simulink model "SoftRobot_AdaptivePassivity_FaultObserver_Tracking_S3"  (R2021b)
settings: Solver=FixedStepAuto  StartTime=0.0  StopTime=30  FixedStep=0.001  RelTol=1e-3  EnableMultiTasking=on
libraries: simulink x3
(part 2 of 2)

== matlab function SoftRobot_AdaptivePassivity_FaultObserver_Tracking_S3/Sliding mode variable//LIP form//Adaptation law ==
  data: Y output; q input; q_dot input; q_des input; theta_hat_dot output; q_dot_des input; q_dotdot_des input; lambda input; adaptation_rate input; r output
function [Y,theta_hat_dot,r] = fcn(q,q_dot,q_des,q_dot_des,q_dotdot_des,lambda,adaptation_rate)

l1=0.067;
l2=0.077;

q1 = q(1);
q2 = q(2);
q_dot1 = q_dot(1);
q_dot2 = q_dot(2);

v = q_dot_des-lambda*(q-q_des);
v1 = v(1);
v2 = v(2);

v_dot = q_dotdot_des-lambda*(q_dot-q_dot_des);
v_dot1 = v_dot(1);
v_dot2 = v_dot(2);

Y1 = [((981*l1*q2*sin(q1))/200 - (981*l1*q1*q2*cos(q1))/200)/(q1^2*q2) - v1*((q_dot2*((2*((l1^2*q2^2)/2 + (l1^2*q1^2*q2^2)/4 - (l1^2*q2^2*cos(q1))/2 - (l1^2*q1*q2^2*sin(q1))/2))/(q1^4*q2^3) - (l1^2*q2 + (l1^2*q1^2*q2)/2 - l1^2*q2*cos(q1) - l1^2*q1*q2*sin(q1))/(q1^4*q2^2)))/2 - (q_dot1*(((l1^2*q1*q2^2)/2 - (l1^2*q1*q2^2*cos(q1))/2)/(q1^4*q2^2) - (4*((l1^2*q2^2)/2 + (l1^2*q1^2*q2^2)/4 - (l1^2*q2^2*cos(q1))/2 - (l1^2*q1*q2^2*sin(q1))/2))/(q1^5*q2^2)))/2) + (v_dot1*((l1^2*q2^2)/2 + (l1^2*q1^2*q2^2)/4 - (l1^2*q2^2*cos(q1))/2 - (l1^2*q1*q2^2*sin(q1))/2))/(q1^4*q2^2), ((981*l1*q2*sin(q1))/100 - (981*l1*q1*q2*cos(q1))/100)/(q1^2*q2) - v1*((q_dot2*((2*(2*l1^2*q2^2 + l1^2*q1^2*q2^2 - 2*l1^2*q2^2*cos(q1) - 2*l1^2*q1*q2^2*sin(q1)))/(q1^4*q2^3) - (4*l1^2*q2 + 2*l1^2*q1^2*q2 - 4*l1^2*q2*cos(q1) - 4*l1^2*q1*q2*sin(q1))/(q1^4*q2^2)))/2 - (q_dot1*((2*l1^2*q1*q2^2 - 2*l1^2*q1*q2^2*cos(q1))/(q1^4*q2^2) - (4*(2*l1^2*q2^2 + l1^2*q1^2*q2^2 - 2*l1^2*q2^2*cos(q1) - 2*l1^2*q1*q2^2*sin(q1)))/(q1^5*q2^2)))/2) + (v_dot1*(2*l1^2*q2^2 + l1^2*q1^2*q2^2 - 2*l1^2*q2^2*cos(q1) - 2*l1^2*q1*q2^2*sin(q1)))/(q1^4*q2^2), ((981*l1*q2*sin(q1))/100 - (981*l1*q1*q2*cos(q1))/100)/(q1^2*q2) - v1*((q_dot2*((2*(2*l1^2*q2^2 + l1^2*q1^2*q2^2 - 2*l1^2*q2^2*cos(q1) - 2*l1^2*q1*q2^2*sin(q1)))/(q1^4*q2^3) - (4*l1^2*q2 + 2*l1^2*q1^2*q2 - 4*l1^2*q2*cos(q1) - 4*l1^2*q1*q2*sin(q1))/(q1^4*q2^2)))/2 - (q_dot1*((2*l1^2*q1*q2^2 - 2*l1^2*q1*q2^2*cos(q1))/(q1^4*q2^2) - (4*(2*l1^2*q2^2 + l1^2*q1^2*q2^2 - 2*l1^2*q2^2*cos(q1) - 2*l1^2*q1*q2^2*sin(q1)))/(q1^5*q2^2)))/2) + (v_dot1*(2*l1^2*q2^2 + l1^2*q1^2*q2^2 - 2*l1^2*q2^2*cos(q1) - 2*l1^2*q1*q2^2*sin(q1)))/(q1^4*q2^2), ((981*l1*q2*sin(q1))/100 - (981*l2*q1^2*cos(q1 + q2))/200 + (981*l2*q1^2*cos(q1))/200 - (981*l1*q1*q2*cos(q1))/100)/(q1^2*q2) - v1*((q_dot1*((4*(2*l1^2*q2^2 + (l2^2*q1^4)/2 + l1^2*q1^2*q2^2 - 2*l1^2*q2^2*cos(q1) - (l2^2*q1^4*cos(q2))/2 - 2*l1^2*q1*q2^2*sin(q1) - l1*l2*q1^3*q2 - l1*l2*q1^2*q2*sin(q1 + q2) + l1*l2*q1^3*q2*cos(q2) + l1*l2*q1^2*q2*sin(q1) + l1*l2*q1^2*q2*sin(q2)))/(q1^5*q2^2) - (2*l2^2*q1^3 + 2*l1^2*q1*q2^2 - 2*l2^2*q1^3*cos(q2) - 2*l1^2*q1*q2^2*cos(q1) - 3*l1*l2*q1^2*q2 - l1*l2*q1^2*q2*cos(q1 + q2) + l1*l2*q1^2*q2*cos(q1) + 3*l1*l2*q1^2*q2*cos(q2) - 2*l1*l2*q1*q2*sin(q1 + q2) + 2*l1*l2*q1*q2*sin(q1) + 2*l1*l2*q1*q2*sin(q2))/(q1^4*q2^2)))/2 + (q_dot2*((2*(2*l1^2*q2^2 + (l2^2*q1^4)/2 + l1^2*q1^2*q2^2 - 2*l1^2*q2^2*cos(q1) - (l2^2*q1^4*cos(q2))/2 - 2*l1^2*q1*q2^2*sin(q1) - l1*l2*q1^3*q2 - l1*l2*q1^2*q2*sin(q1 + q2) + l1*l2*q1^3*q2*cos(q2) + l1*l2*q1^2*q2*sin(q1) + l1*l2*q1^2*q2*sin(q2)))/(q1^4*q2^3) - (4*l1^2*q2 - l1*l2*q1^3 + 2*l1^2*q1^2*q2 - 4*l1^2*q2*cos(q1) + (l2^2*q1^4*sin(q2))/2 - l1*l2*q1^2*sin(q1 + q2) + l1*l2*q1^3*cos(q2) + l1*l2*q1^2*sin(q1) + l1*l2*q1^2*sin(q2) - 4*l1^2*q1*q2*sin(q1) - l1*l2*q1^2*q2*cos(q1 + q2) + l1*l2*q1^2*q2*cos(q2) - l1*l2*q1^3*q2*sin(q2))/(q1^4*q2^2)))/2) + (v_dot1*(2*l1^2*q2^2 + (l2^2*q1^4)/2 + l1^2*q1^2*q2^2 - 2*l1^2*q2^2*cos(q1) - (l2^2*q1^4*cos(q2))/2 - 2*l1^2*q1*q2^2*sin(q1) - l1*l2*q1^3*q2 - l1*l2*q1^2*q2*sin(q1 + q2) + l1*l2*q1^3*q2*cos(q2) + l1*l2*q1^2*q2*sin(q1) + l1*l2*q1^2*q2*sin(q2)))/(q1^4*q2^2) - (l2*v2*(2*l2*q1^2*q_dot1 - 4*l1*q_dot2 + 2*l2*q1^2*q_dot2 + 4*l1*q_dot2*cos(q1) + 4*l1*q_dot2*cos(q2) - 4*l1*q_dot2*cos(q1 + q2) - 2*l1*q1*q2*q_dot1 - 2*l1*q2*q_dot1*sin(q1 + q2) - 4*l1*q2*q_dot2*sin(q1 + q2) + 2*l1*q2*q_dot1*sin(q1) - 4*l1*q1*q_dot2*sin(q2) + 2*l1*q2*q_dot1*sin(q2) + 4*l1*q2*q_dot2*sin(q2) + 2*l1*q2^2*q_dot1*cos(q1 + q2) + 2*l1*q2^2*q_dot2*cos(q1 + q2) - 2*l1*q2^2*q_dot1*cos(q2) - 2*l2*q1^2*q_dot1*cos(q2) - 2*l1*q2^2*q_dot2*cos(q2) - 2*l2*q1^2*q_dot2*cos(q2) + 2*l1*q1*q2^2*q_dot1*sin(q2) + 2*l1*q1*q2^2*q_dot2*sin(q2) - l2*q1^2*q2*q_dot1*sin(q2) - l2*q1^2*q2*q_dot2*sin(q2) + 2*l1*q1*q2*q_dot1*cos(q2) + 4*l1*q1*q2*q_dot2*cos(q2)))/(4*q1^2*q2^3) - (l2*v_dot2*(2*l1 + 2*l1*cos(q1 + q2) - l2*q1^2 - 2*l1*cos(q1) - 2*l1*cos(q2) + 2*l1*q1*sin(q2) - 2*l1*q2*sin(q2) + l2*q1^2*cos(q2) + 2*l1*q2*sin(q1 + q2) - 2*l1*q1*q2*cos(q2)))/(4*q1^2*q2^2), ((981*l1*q2*sin(q1))/100 - (981*l2*q1^2*cos(q1 + q2))/100 + (981*l2*q1^2*cos(q1))/100 - (981*l1*q1*q2*cos(q1))/100)/(q1^2*q2) - v1*((q_dot1*((4*(2*l1^2*q2^2 + 2*l2^2*q1^4 + l1^2*q1^2*q2^2 - 2*l1^2*q2^2*cos(q1) - 2*l2^2*q1^4*cos(q2) - 2*l1^2*q1*q2^2*sin(q1) - 2*l1*l2*q1^3*q2 - 2*l1*l2*q1^2*q2*sin(q1 + q2) + 2*l1*l2*q1^3*q2*cos(q2) + 2*l1*l2*q1^2*q2*sin(q1) + 2*l1*l2*q1^2*q2*sin(q2)))/(q1^5*q2^2) - (8*l2^2*q1^3 + 2*l1^2*q1*q2^2 - 8*l2^2*q1^3*cos(q2) - 2*l1^2*q1*q2^2*cos(q1) - 6*l1*l2*q1^2*q2 - 2*l1*l2*q1^2*q2*cos(q1 + q2) + 2*l1*l2*q1^2*q2*cos(q1) + 6*l1*l2*q1^2*q2*cos(q2) - 4*l1*l2*q1*q2*sin(q1 + q2) + 4*l1*l2*q1*q2*sin(q1) + 4*l1*l2*q1*q2*sin(q2))/(q1^4*q2^2)))/2 + (q_dot2*((2*(2*l1^2*q2^2 + 2*l2^2*q1^4 + l1^2*q1^2*q2^2 - 2*l1^2*q2^2*cos(q1) - 2*l2^2*q1^4*cos(q2) - 2*l1^2*q1*q2^2*sin(q1) - 2*l1*l2*q1^3*q2 - 2*l1*l2*q1^2*q2*sin(q1 + q2) + 2*l1*l2*q1^3*q2*cos(q2) + 2*l1*l2*q1^2*q2*sin(q1) + 2*l1*l2*q1^2*q2*sin(q2)))/(q1^4*q2^3) - (4*l1^2*q2 - 2*l1*l2*q1^3 + 2*l1^2*q1^2*q2 - 4*l1^2*q2*cos(q1) + 2*l2^2*q1^4*sin(q2) - 2*l1*l2*q1^2*sin(q1 + q2) + 2*l1*l2*q1^3*cos(q2) + 2*l1*l2*q1^2*sin(q1) + 2*l1*l2*q1^2*sin(q2) - 4*l1^2*q1*q2*sin(q1) - 2*l1*l2*q1^2*q2*cos(q1 + q2) + 2*l1*l2*q1^2*q2*cos(q2) - 2*l1*l2*q1^3*q2*sin(q2))/(q1^4*q2^2)))/2) + (v_dot1*(2*l1^2*q2^2 + 2*l2^2*q1^4 + l1^2*q1^2*q2^2 - 2*l1^2*q2^2*cos(q1) - 2*l2^2*q1^4*cos(q2) - 2*l1^2*q1*q2^2*sin(q1) - 2*l1*l2*q1^3*q2 - 2*l1*l2*q1^2*q2*sin(q1 + q2) + 2*l1*l2*q1^3*q2*cos(q2) + 2*l1*l2*q1^2*q2*sin(q1) + 2*l1*l2*q1^2*q2*sin(q2)))/(q1^4*q2^2) - (l2*v2*(8*l2*q1^2*q_dot1 - 8*l1*q_dot2 + 8*l2*q1^2*q_dot2 + 8*l1*q_dot2*cos(q1) + 8*l1*q_dot2*cos(q2) - 8*l1*q_dot2*cos(q1 + q2) - 4*l1*q1*q2*q_dot1 - 4*l1*q2*q_dot1*sin(q1 + q2) - 8*l1*q2*q_dot2*sin(q1 + q2) + 4*l1*q2*q_dot1*sin(q1) - 8*l1*q1*q_dot2*sin(q2) + 4*l1*q2*q_dot1*sin(q2) + 8*l1*q2*q_dot2*sin(q2) + 4*l1*q2^2*q_dot1*cos(q1 + q2) + 4*l1*q2^2*q_dot2*cos(q1 + q2) - 4*l1*q2^2*q_dot1*cos(q2) - 8*l2*q1^2*q_dot1*cos(q2) - 4*l1*q2^2*q_dot2*cos(q2) - 8*l2*q1^2*q_dot2*cos(q2) + 4*l1*q1*q2^2*q_dot1*sin(q2) + 4*l1*q1*q2^2*q_dot2*sin(q2) - 4*l2*q1^2*q2*q_dot1*sin(q2) - 4*l2*q1^2*q2*q_dot2*sin(q2) + 4*l1*q1*q2*q_dot1*cos(q2) + 8*l1*q1*q2*q_dot2*cos(q2)))/(4*q1^2*q2^3) - (l2*v_dot2*(4*l1 + 4*l1*cos(q1 + q2) - 4*l2*q1^2 - 4*l1*cos(q1) - 4*l1*cos(q2) + 4*l1*q1*sin(q2) - 4*l1*q2*sin(q2) + 4*l2*q1^2*cos(q2) + 4*l1*q2*sin(q1 + q2) - 4*l1*q1*q2*cos(q2)))/(4*q1^2*q2^2), q1, v1];
Y2 = [(q_dot2*v2*((l2^2*(2*cos(q2) + 2*q2*sin(q2) - q2^2 - 2))/q2^5 + (l2^2*(2*q2 - 2*q2*cos(q2)))/(4*q2^4)))/2 - (981*l2*(sin(q1) - sin(q1 + q2) + q2*cos(q1 + q2)))/(200*q2^2) - (l2^2*v_dot2*(2*cos(q2) + 2*q2*sin(q2) - q2^2 - 2))/(4*q2^4) - (l2*v_dot1*(2*l1 + 2*l1*cos(q1 + q2) - l2*q1^2 - 2*l1*cos(q1) - 2*l1*cos(q2) + 2*l1*q1*sin(q2) - 2*l1*q2*sin(q2) + l2*q1^2*cos(q2) + 2*l1*q2*sin(q1 + q2) - 2*l1*q1*q2*cos(q2)))/(4*q1^2*q2^2) + (l2*q_dot1*v1*(4*l1*q2 + 2*l2*q1^3 - 2*l1*q1^2*q2 - 4*l1*q2*cos(q1) - 4*l1*q2*cos(q2) + 4*l1*q2^2*sin(q1 + q2) - 2*l2*q1^3*cos(q2) - 4*l1*q2^2*sin(q2) + 4*l1*q2*cos(q1 + q2) + 2*l1*q1^2*q2^2*sin(q2) + 4*l1*q1*q2*sin(q2) - 4*l1*q1*q2^2*cos(q2) + 2*l1*q1^2*q2*cos(q2) - l2*q1^3*q2*sin(q2)))/(4*q1^3*q2^3), (q_dot2*v2*((4*l2^2*(2*cos(q2) + 2*q2*sin(q2) - q2^2 - 2))/q2^5 + (l2^2*(2*q2 - 2*q2*cos(q2)))/q2^4))/2 - (981*l2*(sin(q1) - sin(q1 + q2) + q2*cos(q1 + q2)))/(100*q2^2) - (l2^2*v_dot2*(2*cos(q2) + 2*q2*sin(q2) - q2^2 - 2))/q2^4 - (l2*v_dot1*(4*l1 + 4*l1*cos(q1 + q2) - 4*l2*q1^2 - 4*l1*cos(q1) - 4*l1*cos(q2) + 4*l1*q1*sin(q2) - 4*l1*q2*sin(q2) + 4*l2*q1^2*cos(q2) + 4*l1*q2*sin(q1 + q2) - 4*l1*q1*q2*cos(q2)))/(4*q1^2*q2^2) + (l2*q_dot1*v1*(8*l1*q2 + 8*l2*q1^3 - 4*l1*q1^2*q2 - 8*l1*q2*cos(q1) - 8*l1*q2*cos(q2) + 8*l1*q2^2*sin(q1 + q2) - 8*l2*q1^3*cos(q2) - 8*l1*q2^2*sin(q2) + 8*l1*q2*cos(q1 + q2) + 4*l1*q1^2*q2^2*sin(q2) + 8*l1*q1*q2*sin(q2) - 8*l1*q1*q2^2*cos(q2) + 4*l1*q1^2*q2*cos(q2) - 4*l2*q1^3*q2*sin(q2)))/(4*q1^3*q2^3), q2, v2];
Y = blkdiag(Y1,Y2);

% Y=[ -(l1*(981*q1^4*cos(q1) - 981*q1^3*sin(q1) - 50*l1*q1^3*v_dot1 - 100*l1*q1*v_dot1 + 200*l1*q_dot1*v1 + 50*l1*q1^2*q_dot1*v1 + 100*l1*q1*v_dot1*cos(q1) - 200*l1*q_dot1*v1*cos(q1) + 100*l1*q1^2*v_dot1*sin(q1) - 200*l1*q1*q_dot1*v1*sin(q1) + 50*l1*q1^2*q_dot1*v1*cos(q1)))/(200*q1^5), -(l1*(981*q1^4*cos(q1) - 981*q1^3*sin(q1) - 100*l1*q1^3*v_dot1 - 200*l1*q1*v_dot1 + 400*l1*q_dot1*v1 + 100*l1*q1^2*q_dot1*v1 + 200*l1*q1*v_dot1*cos(q1) - 400*l1*q_dot1*v1*cos(q1) + 200*l1*q1^2*v_dot1*sin(q1) - 400*l1*q1*q_dot1*v1*sin(q1) + 100*l1*q1^2*q_dot1*v1*cos(q1)))/(100*q1^5), -(l1*(981*q1^4*cos(q1) - 981*q1^3*sin(q1) - 100*l1*q1^3*v_dot1 - 200*l1*q1*v_dot1 + 400*l1*q_dot1*v1 + 100*l1*q1^2*q_dot1*v1 + 200*l1*q1*v_dot1*cos(q1) - 400*l1*q_dot1*v1*cos(q1) + 200*l1*q1^2*v_dot1*sin(q1) - 400*l1*q1*q_dot1*v1*sin(q1) + 100*l1*q1^2*q_dot1*v1*cos(q1)))/(100*q1^5), (1962*l1*q2*sin(q1) - 981*l2*q1^2*cos(q1 + q2) + 981*l2*q1^2*cos(q1) - 1962*l1*q1*q2*cos(q1))/(200*q1^2*q2) + (v_dot1*(2*l1^2*q2^2 + (l2^2*q1^4)/2 + l1^2*q1^2*q2^2 - 2*l1^2*q2^2*cos(q1) - (l2^2*q1^4*cos(q2))/2 - 2*l1^2*q1*q2^2*sin(q1) - l1*l2*q1^3*q2 - l1*l2*q1^2*q2*sin(q1 + q2) + l1*l2*q1^3*q2*cos(q2) + l1*l2*q1^2*q2*sin(q1) + l1*l2*q1^2*q2*sin(q2)))/(q1^4*q2^2) - (l2*v2*(4*l2*q1^2*q_dot1 - 4*l1*q_dot2 + 2*l2*q1^2*q_dot2 + 4*l1*q_dot2*cos(q1) + 4*l1*q_dot2*cos(q2) - 4*l1*q_dot2*cos(q1 + q2) - 4*l1*q1*q2*q_dot1 - 4*l1*q2*q_dot1*sin(q1 + q2) - 4*l1*q2*q_dot2*sin(q1 + q2) + 4*l1*q2*q_dot1*sin(q1) - 4*l1*q1*q_dot2*sin(q2) + 4*l1*q2*q_dot1*sin(q2) + 4*l1*q2*q_dot2*sin(q2) + 4*l1*q2^2*q_dot1*cos(q1 + q2) + 2*l1*q2^2*q_dot2*cos(q1 + q2) - 4*l1*q2^2*q_dot1*cos(q2) - 4*l2*q1^2*q_dot1*cos(q2) - 2*l1*q2^2*q_dot2*cos(q2) - 2*l2*q1^2*q_dot2*cos(q2) + 4*l1*q1*q2^2*q_dot1*sin(q2) + 2*l1*q1*q2^2*q_dot2*sin(q2) - 2*l2*q1^2*q2*q_dot1*sin(q2) - l2*q1^2*q2*q_dot2*sin(q2) + 4*l1*q1*q2*q_dot1*cos(q2) + 4*l1*q1*q2*q_dot2*cos(q2)))/(4*q1^2*q2^3) - (l2*v_dot2*(2*l1 + 2*l1*cos(q1 + q2) - l2*q1^2 - 2*l1*cos(q1) - 2*l1*cos(q2) + 2*l1*q1*sin(q2) - 2*l1*q2*sin(q2) + l2*q1^2*cos(q2) + 2*l1*q2*sin(q1 + q2) - 2*l1*q1*q2*cos(q2)))/(4*q1^2*q2^2) - (l1*q_dot1*v1*(8*l1*q2 - l2*q1^3 + 2*l1*q1^2*q2 - 8*l1*q2*cos(q1) + l2*q1^3*cos(q1 + q2) - 2*l2*q1^2*sin(q1 + q2) - l2*q1^3*cos(q1) + l2*q1^3*cos(q2) + 2*l2*q1^2*sin(q1) + 2*l2*q1^2*sin(q2) - 8*l1*q1*q2*sin(q1) + 2*l1*q1^2*q2*cos(q1)))/(2*q1^5*q2), (981*l1*q2*sin(q1) - 981*l2*q1^2*cos(q1 + q2) + 981*l2*q1^2*cos(q1) - 981*l1*q1*q2*cos(q1))/(100*q1^2*q2) + (v_dot1*(2*l1^2*q2^2 + 2*l2^2*q1^4 + l1^2*q1^2*q2^2 - 2*l1^2*q2^2*cos(q1) - 2*l2^2*q1^4*cos(q2) - 2*l1^2*q1*q2^2*sin(q1) - 2*l1*l2*q1^3*q2 - 2*l1*l2*q1^2*q2*sin(q1 + q2) + 2*l1*l2*q1^3*q2*cos(q2) + 2*l1*l2*q1^2*q2*sin(q1) + 2*l1*l2*q1^2*q2*sin(q2)))/(q1^4*q2^2) - (l2*v2*(4*l2*q1^2*q_dot1 - 2*l1*q_dot2 + 2*l2*q1^2*q_dot2 + 2*l1*q_dot2*cos(q1) + 2*l1*q_dot2*cos(q2) - 2*l1*q_dot2*cos(q1 + q2) - 2*l1*q1*q2*q_dot1 - 2*l1*q2*q_dot1*sin(q1 + q2) - 2*l1*q2*q_dot2*sin(q1 + q2) + 2*l1*q2*q_dot1*sin(q1) - 2*l1*q1*q_dot2*sin(q2) + 2*l1*q2*q_dot1*sin(q2) + 2*l1*q2*q_dot2*sin(q2) + 2*l1*q2^2*q_dot1*cos(q1 + q2) + l1*q2^2*q_dot2*cos(q1 + q2) - 2*l1*q2^2*q_dot1*cos(q2) - 4*l2*q1^2*q_dot1*cos(q2) - l1*q2^2*q_dot2*cos(q2) - 2*l2*q1^2*q_dot2*cos(q2) + 2*l1*q1*q2^2*q_dot1*sin(q2) + l1*q1*q2^2*q_dot2*sin(q2) - 2*l2*q1^2*q2*q_dot1*sin(q2) - l2*q1^2*q2*q_dot2*sin(q2) + 2*l1*q1*q2*q_dot1*cos(q2) + 2*l1*q1*q2*q_dot2*cos(q2)))/(q1^2*q2^3) - (l2*v_dot2*(4*l1 + 4*l1*cos(q1 + q2) - 4*l2*q1^2 - 4*l1*cos(q1) - 4*l1*cos(q2) + 4*l1*q1*sin(q2) - 4*l1*q2*sin(q2) + 4*l2*q1^2*cos(q2) + 4*l1*q2*sin(q1 + q2) - 4*l1*q1*q2*cos(q2)))/(4*q1^2*q2^2) - (l1*q_dot1*v1*(4*l1*q2 - l2*q1^3 + l1*q1^2*q2 - 4*l1*q2*cos(q1) + l2*q1^3*cos(q1 + q2) - 2*l2*q1^2*sin(q1 + q2) - l2*q1^3*cos(q1) + l2*q1^3*cos(q2) + 2*l2*q1^2*sin(q1) + 2*l2*q1^2*sin(q2) - 4*l1*q1*q2*sin(q1) + l1*q1^2*q2*cos(q1)))/(q1^5*q2), q1,  0, v1,      0
%                                                                                                                                                                                                                                                                                                                   0,                                                                                                                                                                                                                                                                                                                     0,                                                                                                                                                                                                                                                                                                                     0,                                                                                                                                                                                                                                                                                                                                                                                                                                                                                                                                                                                                                                                                                                                                                                                  (l2*q_dot1*v1*(4*l1*q2 + 2*l2*q1^3 - 2*l1*q1^2*q2 - 4*l1*q2*cos(q1) - 4*l1*q2*cos(q2) + 4*l1*q2^2*sin(q1 + q2) - 2*l2*q1^3*cos(q2) - 4*l1*q2^2*sin(q2) + 4*l1*q2*cos(q1 + q2) + 2*l1*q1^2*q2^2*sin(q2) + 4*l1*q1*q2*sin(q2) - 4*l1*q1*q2^2*cos(q2) + 2*l1*q1^2*q2*cos(q2) - l2*q1^3*q2*sin(q2)))/(4*q1^3*q2^3) - (l2^2*v_dot2*(2*cos(q2) + 2*q2*sin(q2) - q2^2 - 2))/(4*q2^4) - (l2*v_dot1*(2*l1 + 2*l1*cos(q1 + q2) - l2*q1^2 - 2*l1*cos(q1) - 2*l1*cos(q2) + 2*l1*q1*sin(q2) - 2*l1*q2*sin(q2) + l2*q1^2*cos(q2) + 2*l1*q2*sin(q1 + q2) - 2*l1*q1*q2*cos(q2)))/(4*q1^2*q2^2) - (l2^2*q_dot2*v2*(q2^2*cos(q2) - 4*cos(q2) - 4*q2*sin(q2) + q2^2 + 4))/(4*q2^5) - (981*l2*(sin(q1) - sin(q1 + q2) + q2*cos(q1 + q2)))/(200*q2^2),                                                                                                                                                                                                                                                                                                                                                                                                                                                                                                                                                                                                                                                                                                                                                                                        (l2*q_dot1*v1*(2*l1*q2 + 2*l2*q1^3 - l1*q1^2*q2 - 2*l1*q2*cos(q1) - 2*l1*q2*cos(q2) + 2*l1*q2^2*sin(q1 + q2) - 2*l2*q1^3*cos(q2) - 2*l1*q2^2*sin(q2) + 2*l1*q2*cos(q1 + q2) + l1*q1^2*q2^2*sin(q2) + 2*l1*q1*q2*sin(q2) - 2*l1*q1*q2^2*cos(q2) + l1*q1^2*q2*cos(q2) - l2*q1^3*q2*sin(q2)))/(q1^3*q2^3) - (l2^2*v_dot2*(2*cos(q2) + 2*q2*sin(q2) - q2^2 - 2))/q2^4 - (l2*v_dot1*(4*l1 + 4*l1*cos(q1 + q2) - 4*l2*q1^2 - 4*l1*cos(q1) - 4*l1*cos(q2) + 4*l1*q1*sin(q2) - 4*l1*q2*sin(q2) + 4*l2*q1^2*cos(q2) + 4*l1*q2*sin(q1 + q2) - 4*l1*q1*q2*cos(q2)))/(4*q1^2*q2^2) - (l2^2*q_dot2*v2*(q2^2*cos(q2) - 4*cos(q2) - 4*q2*sin(q2) + q2^2 + 4))/q2^5 - (981*l2*(sin(q1) - sin(q1 + q2) + q2*cos(q1 + q2)))/(100*q2^2),  0, q2,      0, v2];
% 
r = [q_dot1;q_dot2]-v;

theta_hat_dot = -adaptation_rate*Y'*r;

== matlab function SoftRobot_AdaptivePassivity_FaultObserver_Tracking_S3/Control law with observed fault ==
  data: Y input; theta_hat input; r input; torque output; K input; Xi_hat input
function torque = fcn(Y,theta_hat,r,K,Xi_hat)

torque = Y*theta_hat-K*r + Xi_hat;

== matlab function SoftRobot_AdaptivePassivity_FaultObserver_Tracking_S3/Soft robot dynamic model ==
  data: q_dotdot output; M output; M_inv output; N_bar output; q input; q_dot input; torque input
function [q_dotdot, M, M_inv, N_bar] = fcn(q, q_dot, torque)
mu1 = 0.02/3;
mu2 = 0.02/3;
mu3 = 0;
mu4 = 0.02/3;
l1 = 0.067;
l2 = 0.077;
mu5 = 0.0251/3;
mu6 = 0.0251/3;
mu7 = 0;
mu8 = 0.0251/3;

q1 = q(1);
q2 = q(2);
qdot1 = q_dot(1);
qdot2 = q_dot(2);

M=[ (0.25*(2.0*l1^2*mu2*q2^2 + 8.0*l1^2*mu4*q2^2 + 8.0*l1^2*mu5*q2^2 + 8.0*l1^2*mu6*q2^2 + 8.0*l1^2*mu8*q2^2 + 2.0*l2^2*mu6*q1^4 + 8.0*l2^2*mu8*q1^4 + l1^2*mu2*q1^2*q2^2 + 4.0*l1^2*mu4*q1^2*q2^2 + 4.0*l1^2*mu5*q1^2*q2^2 + 4.0*l1^2*mu6*q1^2*q2^2 + 4.0*l1^2*mu8*q1^2*q2^2 - 2.0*l1^2*mu2*q2^2*cos(q1) - 8.0*l1^2*mu4*q2^2*cos(q1) - 8.0*l1^2*mu5*q2^2*cos(q1) - 8.0*l1^2*mu6*q2^2*cos(q1) - 8.0*l1^2*mu8*q2^2*cos(q1) - 2.0*l2^2*mu6*q1^4*cos(q2) - 8.0*l2^2*mu8*q1^4*cos(q2) - 2.0*l1^2*mu2*q1*q2^2*sin(q1) - 8.0*l1^2*mu4*q1*q2^2*sin(q1) - 8.0*l1^2*mu5*q1*q2^2*sin(q1) - 8.0*l1^2*mu6*q1*q2^2*sin(q1) - 8.0*l1^2*mu8*q1*q2^2*sin(q1) - 4.0*l1*l2*mu6*q1^3*q2 - 8.0*l1*l2*mu8*q1^3*q2 - 4.0*l1*l2*mu6*q1^2*q2*sin(q1 + q2) - 8.0*l1*l2*mu8*q1^2*q2*sin(q1 + q2) + 4.0*l1*l2*mu6*q1^3*q2*cos(q2) + 8.0*l1*l2*mu8*q1^3*q2*cos(q2) + 4.0*l1*l2*mu6*q1^2*q2*sin(q1) + 4.0*l1*l2*mu6*q1^2*q2*sin(q2) + 8.0*l1*l2*mu8*q1^2*q2*sin(q1) + 8.0*l1*l2*mu8*q1^2*q2*sin(q2)))/(q1^4*q2^2), -(0.25*l2*(2.0*l1*mu6 + 4.0*l1*mu8 - 1.0*l2*mu6*q1^2 - 4.0*l2*mu8*q1^2 - 2.0*l1*mu6*cos(q1) - 2.0*l1*mu6*cos(q2) - 4.0*l1*mu8*cos(q1) - 4.0*l1*mu8*cos(q2) + 2.0*l1*mu6*cos(q1 + q2) + 4.0*l1*mu8*cos(q1 + q2) + 2.0*l1*mu6*q2*sin(q1 + q2) + 4.0*l1*mu8*q2*sin(q1 + q2) + 2.0*l1*mu6*q1*sin(q2) - 2.0*l1*mu6*q2*sin(q2) + 4.0*l1*mu8*q1*sin(q2) - 4.0*l1*mu8*q2*sin(q2) + l2*mu6*q1^2*cos(q2) + 4.0*l2*mu8*q1^2*cos(q2) - 2.0*l1*mu6*q1*q2*cos(q2) - 4.0*l1*mu8*q1*q2*cos(q2)))/(q1^2*q2^2)
                                                                                                                                                                                                                                                                                                                                                                                                                                                                                     -(0.25*l2*(2.0*l1*mu6 + 4.0*l1*mu8 - 1.0*l2*mu6*q1^2 - 4.0*l2*mu8*q1^2 - 2.0*l1*mu6*cos(q1) - 2.0*l1*mu6*cos(q2) - 4.0*l1*mu8*cos(q1) - 4.0*l1*mu8*cos(q2) + 2.0*l1*mu6*cos(q1 + q2) + 4.0*l1*mu8*cos(q1 + q2) + 2.0*l1*mu6*q2*sin(q1 + q2) + 4.0*l1*mu8*q2*sin(q1 + q2) + 2.0*l1*mu6*q1*sin(q2) - 2.0*l1*mu6*q2*sin(q2) + 4.0*l1*mu8*q1*sin(q2) - 4.0*l1*mu8*q2*sin(q2) + l2*mu6*q1^2*cos(q2) + 4.0*l2*mu8*q1^2*cos(q2) - 2.0*l1*mu6*q1*q2*cos(q2) - 4.0*l1*mu8*q1*q2*cos(q2)))/(q1^2*q2^2),                                                                                                                                                                                                                                                                                                                                                                                                            -(0.25*l2^2*(mu6 + 4.0*mu8)*(2.0*cos(q2) + 2.0*q2*sin(q2) - 1.0*q2^2 - 2.0))/q2^4];

C_q=[-(0.5*(2.0*l1^2*mu2*q2^3*qdot1^2 + 8.0*l1^2*mu4*q2^3*qdot1^2 + 8.0*l1^2*mu5*q2^3*qdot1^2 + 8.0*l1^2*mu6*q2^3*qdot1^2 + 8.0*l1^2*mu8*q2^3*qdot1^2 + l2^2*mu6*q1^5*qdot2^2 + 4.0*l2^2*mu8*q1^5*qdot2^2 + 0.5*l1^2*mu2*q1^2*q2^3*qdot1^2 + 2.0*l1^2*mu4*q1^2*q2^3*qdot1^2 + 2.0*l1^2*mu5*q1^2*q2^3*qdot1^2 + 2.0*l1^2*mu6*q1^2*q2^3*qdot1^2 + 2.0*l1^2*mu8*q1^2*q2^3*qdot1^2 - 2.0*l1^2*mu2*q2^3*qdot1^2*cos(q1) - 8.0*l1^2*mu4*q2^3*qdot1^2*cos(q1) - 8.0*l1^2*mu5*q2^3*qdot1^2*cos(q1) - 8.0*l1^2*mu6*q2^3*qdot1^2*cos(q1) - 8.0*l1^2*mu8*q2^3*qdot1^2*cos(q1) - 1.0*l2^2*mu6*q1^5*qdot2^2*cos(q2) - 4.0*l2^2*mu8*q1^5*qdot2^2*cos(q2) - 2.0*l1*l2*mu6*q1^3*qdot2^2 - 4.0*l1*l2*mu8*q1^3*qdot2^2 + 2.0*l2^2*mu6*q1^5*qdot1*qdot2 + 8.0*l2^2*mu8*q1^5*qdot1*qdot2 - 1.0*l1*l2*mu6*q1^3*q2^2*qdot1^2 - 2.0*l1*l2*mu8*q1^3*q2^2*qdot1^2 + 2.0*l1*l2*mu6*q1^3*qdot2^2*cos(q1) + 2.0*l1*l2*mu6*q1^3*qdot2^2*cos(q2) + 4.0*l1*l2*mu8*q1^3*qdot2^2*cos(q1) + 4.0*l1*l2*mu8*q1^3*qdot2^2*cos(q2) - 2.0*l2^2*mu6*q1^5*qdot1*qdot2*cos(q2) - 8.0*l2^2*mu8*q1^5*qdot1*qdot2*cos(q2) - 2.0*l1*l2*mu6*q1^4*qdot2^2*sin(q2) - 4.0*l1*l2*mu8*q1^4*qdot2^2*sin(q2) - 2.0*l1^2*mu2*q1*q2^3*qdot1^2*sin(q1) - 8.0*l1^2*mu4*q1*q2^3*qdot1^2*sin(q1) - 8.0*l1^2*mu5*q1*q2^3*qdot1^2*sin(q1) - 8.0*l1^2*mu6*q1*q2^3*qdot1^2*sin(q1) - 8.0*l1^2*mu8*q1*q2^3*qdot1^2*sin(q1) - 0.5*l2^2*mu6*q1^5*q2*qdot2^2*sin(q2) - 2.0*l2^2*mu8*q1^5*q2*qdot2^2*sin(q2) + 0.5*l1^2*mu2*q1^2*q2^3*qdot1^2*cos(q1) + 2.0*l1^2*mu4*q1^2*q2^3*qdot1^2*cos(q1) + 2.0*l1^2*mu5*q1^2*q2^3*qdot1^2*cos(q1) + 2.0*l1^2*mu6*q1^2*q2^3*qdot1^2*cos(q1) + 2.0*l1^2*mu8*q1^2*q2^3*qdot1^2*cos(q1) - 2.0*l1*l2*mu6*q1^3*qdot2^2*cos(q1 + q2) - 4.0*l1*l2*mu8*q1^3*qdot2^2*cos(q1 + q2) - 2.0*l1*l2*mu6*q1^3*q2*qdot2^2*sin(q1 + q2) - 4.0*l1*l2*mu8*q1^3*q2*qdot2^2*sin(q1 + q2) + 2.0*l1*l2*mu6*q1^4*q2*qdot2^2*cos(q2) + 4.0*l1*l2*mu8*q1^4*q2*qdot2^2*cos(q2) + 2.0*l1*l2*mu6*q1^3*q2*qdot2^2*sin(q2) + 4.0*l1*l2*mu8*q1^3*q2*qdot2^2*sin(q2) - 1.0*l2^2*mu6*q1^5*q2*qdot1*qdot2*sin(q2) - 4.0*l2^2*mu8*q1^5*q2*qdot1*qdot2*sin(q2) + l1*l2*mu6*q1^3*q2^2*qdot1^2*cos(q1 + q2) + l1*l2*mu6*q1^3*q2^2*qdot2^2*cos(q1 + q2) + 2.0*l1*l2*mu8*q1^3*q2^2*qdot1^2*cos(q1 + q2) + 2.0*l1*l2*mu8*q1^3*q2^2*qdot2^2*cos(q1 + q2) - 2.0*l1*l2*mu6*q1^4*q2*qdot1*qdot2 - 4.0*l1*l2*mu8*q1^4*q2*qdot1*qdot2 - 2.0*l1*l2*mu6*q1^2*q2^2*qdot1^2*sin(q1 + q2) - 4.0*l1*l2*mu8*q1^2*q2^2*qdot1^2*sin(q1 + q2) - 1.0*l1*l2*mu6*q1^3*q2^2*qdot1^2*cos(q1) + l1*l2*mu6*q1^3*q2^2*qdot1^2*cos(q2) - 1.0*l1*l2*mu6*q1^3*q2^2*qdot2^2*cos(q2) - 2.0*l1*l2*mu8*q1^3*q2^2*qdot1^2*cos(q1) + 2.0*l1*l2*mu8*q1^3*q2^2*qdot1^2*cos(q2) - 2.0*l1*l2*mu8*q1^3*q2^2*qdot2^2*cos(q2) + 2.0*l1*l2*mu6*q1^2*q2^2*qdot1^2*sin(q1) + 2.0*l1*l2*mu6*q1^2*q2^2*qdot1^2*sin(q2) + 4.0*l1*l2*mu8*q1^2*q2^2*qdot1^2*sin(q1) + 4.0*l1*l2*mu8*q1^2*q2^2*qdot1^2*sin(q2) + l1*l2*mu6*q1^4*q2^2*qdot2^2*sin(q2) + 2.0*l1*l2*mu8*q1^4*q2^2*qdot2^2*sin(q2) + 2.0*l1*l2*mu6*q1^4*q2^2*qdot1*qdot2*sin(q2) + 4.0*l1*l2*mu8*q1^4*q2^2*qdot1*qdot2*sin(q2) - 2.0*l1*l2*mu6*q1^3*q2*qdot1*qdot2*sin(q1 + q2) - 4.0*l1*l2*mu8*q1^3*q2*qdot1*qdot2*sin(q1 + q2) + 2.0*l1*l2*mu6*q1^4*q2*qdot1*qdot2*cos(q2) + 4.0*l1*l2*mu8*q1^4*q2*qdot1*qdot2*cos(q2) + 2.0*l1*l2*mu6*q1^3*q2*qdot1*qdot2*sin(q1) + 2.0*l1*l2*mu6*q1^3*q2*qdot1*qdot2*sin(q2) + 4.0*l1*l2*mu8*q1^3*q2*qdot1*qdot2*sin(q1) + 4.0*l1*l2*mu8*q1^3*q2*qdot1*qdot2*sin(q2) + 2.0*l1*l2*mu6*q1^3*q2^2*qdot1*qdot2*cos(q1 + q2) + 4.0*l1*l2*mu8*q1^3*q2^2*qdot1*qdot2*cos(q1 + q2) - 2.0*l1*l2*mu6*q1^3*q2^2*qdot1*qdot2*cos(q2) - 4.0*l1*l2*mu8*q1^3*q2^2*qdot1*qdot2*cos(q2)))/(q1^5*q2^3)
                                                                                                                                                                                                                                                                                                                                                                                                                                                                                                                                                                                                                                                                                                                                                                                                                                                                                                                                                                                                                                                                                                                                                                                                                                                                                                                                                                                                                                                                                                                                                                                                                                                                                                                                                                                                                                                                                                                                                                                                                                                                                                                                                                                                                                                     -(0.25*l2*(4.0*l2*mu6*q1^3*qdot2^2 - 4.0*l1*mu6*q2^3*qdot1^2 - 8.0*l1*mu8*q2^3*qdot1^2 + 16.0*l2*mu8*q1^3*qdot2^2 - 4.0*l1*mu6*q2^3*qdot1^2*cos(q1 + q2) - 8.0*l1*mu8*q2^3*qdot1^2*cos(q1 + q2) - 4.0*l1*mu6*q2^4*qdot1^2*sin(q1 + q2) - 8.0*l1*mu8*q2^4*qdot1^2*sin(q1 + q2) + 2.0*l1*mu6*q1^2*q2^3*qdot1^2 - 2.0*l2*mu6*q1^3*q2^2*qdot1^2 + 4.0*l1*mu8*q1^2*q2^3*qdot1^2 + l2*mu6*q1^3*q2^2*qdot2^2 - 8.0*l2*mu8*q1^3*q2^2*qdot1^2 + 4.0*l2*mu8*q1^3*q2^2*qdot2^2 + 4.0*l1*mu6*q2^3*qdot1^2*cos(q1) + 4.0*l1*mu6*q2^3*qdot1^2*cos(q2) + 8.0*l1*mu8*q2^3*qdot1^2*cos(q1) - 4.0*l2*mu6*q1^3*qdot2^2*cos(q2) + 8.0*l1*mu8*q2^3*qdot1^2*cos(q2) - 16.0*l2*mu8*q1^3*qdot2^2*cos(q2) + 4.0*l1*mu6*q2^4*qdot1^2*sin(q2) + 8.0*l1*mu8*q2^4*qdot1^2*sin(q2) + 4.0*l1*mu6*q1*q2^4*qdot1^2*cos(q2) + 8.0*l1*mu8*q1*q2^4*qdot1^2*cos(q2) - 4.0*l1*mu6*q1*q2^3*qdot1^2*sin(q2) - 8.0*l1*mu8*q1*q2^3*qdot1^2*sin(q2) - 4.0*l2*mu6*q1^3*q2*qdot2^2*sin(q2) - 16.0*l2*mu8*q1^3*q2*qdot2^2*sin(q2) - 2.0*l1*mu6*q1^2*q2^3*qdot1^2*cos(q2) + 2.0*l2*mu6*q1^3*q2^2*qdot1^2*cos(q2) - 4.0*l1*mu8*q1^2*q2^3*qdot1^2*cos(q2) + l2*mu6*q1^3*q2^2*qdot2^2*cos(q2) + 8.0*l2*mu8*q1^3*q2^2*qdot1^2*cos(q2) + 4.0*l2*mu8*q1^3*q2^2*qdot2^2*cos(q2) - 2.0*l1*mu6*q1^2*q2^4*qdot1^2*sin(q2) + l2*mu6*q1^3*q2^3*qdot1^2*sin(q2) - 4.0*l1*mu8*q1^2*q2^4*qdot1^2*sin(q2) + 4.0*l2*mu8*q1^3*q2^3*qdot1^2*sin(q2)))/(q1^3*q2^5)];
                                                                                                                                                                                                                                                                                                                                                                                                                                                                                                                                                                                                                                                                                                                                                                                                                                                                                                                                                                                                                                                                                                  
G=[-(0.005*(981.0*l2*q1^2*cos(q1 + q2)*conj(mu6) + 1962.0*l2*q1^2*cos(q1 + q2)*conj(mu8) - 981.0*l2*q1^2*conj(mu6)*cos(q1) - 1962.0*l2*q1^2*conj(mu8)*cos(q1) - 981.0*l1*mu2*q2*sin(q1) - 1962.0*l1*q2*conj(mu4)*sin(q1) - 1962.0*l1*q2*conj(mu5)*sin(q1) - 1962.0*l1*q2*conj(mu6)*sin(q1) - 1962.0*l1*q2*conj(mu8)*sin(q1) + 1962.0*l1*q1*q2*conj(mu4)*cos(q1) + 1962.0*l1*q1*q2*conj(mu5)*cos(q1) + 1962.0*l1*q1*q2*conj(mu6)*cos(q1) + 1962.0*l1*q1*q2*conj(mu8)*cos(q1) + 981.0*l1*mu2*q1*q2*cos(q1)))/(q1^2*q2)
                                                                                                                                                                                                                                                                                                                                                                                                                       -(4.905*l2*(conj(mu6) + 2.0*conj(mu8))*(sin(q1) - 1.0*sin(q1 + q2) + q2*cos(q1 + q2)))/q2^2];

K=[0.68,0;0,0.7];
D=[0.0029,0;0,0.003];

q_dotdot=(eye(2)/M)*(torque-K*[q1;q2]-D*[qdot1;qdot2]-C_q-G);
M_inv = eye(2)/M;
N_bar=(eye(2)/M)*(K*[q1;q2]+D*[qdot1;qdot2]+C_q+G);
